simulink model "main"  (R2022a)
settings: Solver=FixedStepDiscrete  StartTime=0.0  StopTime=Inf  FixedStep=(50e-6)-(sim_en*4.995e-5)  RelTol=1e-3  EnableMultiTasking=on
model workspace (MAT data in the model file):
  Param : Simulink.Parameter (value not decoded)
  ac_ok : Simulink.Signal (value not decoded)
  ac_ok_120 : Simulink.Signal (value not decoded)
  bulk_voltage : Simulink.Signal (value not decoded)
  burstduty_integ_max : Simulink.Signal (value not decoded)
  burstduty_integ_min : Simulink.Signal (value not decoded)
  burstduty_ki : Simulink.Signal (value not decoded)
  burstduty_kp : Simulink.Signal (value not decoded)
  calib_ok : Simulink.Signal (value not decoded)
  can_addr1 : Simulink.Signal (value not decoded)
  can_addr2 : Simulink.Signal (value not decoded)
  can_addr3 : Simulink.Signal (value not decoded)
  can_addr4 : Simulink.Signal (value not decoded)
  can_data_rx : Simulink.Signal (value not decoded)
  can_data_tx : Simulink.Signal (value not decoded)
  can_timeout_120 : Simulink.Signal (value not decoded)
  chksum_scircv : Simulink.Signal (value not decoded)
  clllc_en_120 : Simulink.Signal (value not decoded)
  clllc_fault_120 : Simulink.Signal (value not decoded)
  clllc_ok_120 : Simulink.Signal (value not decoded)
  cmpss1h : Simulink.Signal (value not decoded)
  cmpss1l : Simulink.Signal (value not decoded)
  cmpss2h : Simulink.Signal (value not decoded)
  cmpss2l : Simulink.Signal (value not decoded)
  cmpss3h : Simulink.Signal (value not decoded)
  cmpss3l : Simulink.Signal (value not decoded)
  cmpss4h : Simulink.Signal (value not decoded)
  cmpss4l : Simulink.Signal (value not decoded)
  cmpss5h : Simulink.Signal (value not decoded)
  cmpss5l : Simulink.Signal (value not decoded)
  cmpss6h : Simulink.Signal (value not decoded)
  cmpss6l : Simulink.Signal (value not decoded)
  cmpss7h : Simulink.Signal (value not decoded)
  cmpss7l : Simulink.Signal (value not decoded)
  cmpss8h : Simulink.Signal (value not decoded)
  cmpss8l : Simulink.Signal (value not decoded)
  cnt_idle : Simulink.Signal (value not decoded)
  cnt_orps : Simulink.Signal (value not decoded)
  cnt_scircv : Simulink.Signal (value not decoded)
  cnt_scixmt : Simulink.Signal (value not decoded)
  cnt_scixmt_func : Simulink.Signal (value not decoded)
  cnt_temp_mux : Simulink.Signal (value not decoded)
  cnt_vdroop : Simulink.Signal (value not decoded)
  config_ok : Simulink.Signal (value not decoded)
  control_en : Simulink.Signal (value not decoded)
  cp_ready_120 : Simulink.Signal (value not decoded)
  d2d_en : Simulink.Signal (value not decoded)
  dchg_off : Simulink.Signal (value not decoded)
  debug_dacb : Simulink.Signal (value not decoded)
  debug_dacc : Simulink.Signal (value not decoded)
  debug_msg1 : Simulink.Signal (value not decoded)
  debug_msg2 : Simulink.Signal (value not decoded)
  debug_msg3 : Simulink.Signal (value not decoded)
  debug_msg4 : Simulink.Signal (value not decoded)
  debug_msg5 : Simulink.Signal (value not decoded)
  debug_msg6 : Simulink.Signal (value not decoded)
  dir_v2g : Simulink.Signal (value not decoded)
  eoss_llc1 : Simulink.Signal (value not decoded)
  eoss_llc2 : Simulink.Signal (value not decoded)
  eoss_orps : Simulink.Signal (value not decoded)
  fault_ocp : Simulink.Signal (value not decoded)
  fault_otp : Simulink.Signal (value not decoded)
  fault_ovp : Simulink.Signal (value not decoded)
  fut_en : Simulink.Signal (value not decoded)
  fwd_en_120 : Simulink.Signal (value not decoded)
  gain_llc1_sec_idc : Simulink.Signal (value not decoded)
  gain_llc1_temp_sr : Simulink.Signal (value not decoded)
  gain_llc2_sec_idc : Simulink.Signal (value not decoded)
  gain_vbat : Simulink.Signal (value not decoded)
  gain_vbulk : Simulink.Signal (value not decoded)
  gain_vout : Simulink.Signal (value not decoded)
  input_current_phasea : Simulink.Signal (value not decoded)
  input_current_phaseb : Simulink.Signal (value not decoded)
  input_current_phasec : Simulink.Signal (value not decoded)
  input_freq : Simulink.Signal (value not decoded)
  input_power : Simulink.Signal (value not decoded)
  input_voltage_phasea : Simulink.Signal (value not decoded)
  input_voltage_phaseb : Simulink.Signal (value not decoded)
  input_voltage_phasec : Simulink.Signal (value not decoded)
  ishare_arbiter : Simulink.Signal (value not decoded)
  ishare_thresh : Simulink.Signal (value not decoded)
  led_g : Simulink.Signal (value not decoded)
  led_r : Simulink.Signal (value not decoded)
  led_y : Simulink.Signal (value not decoded)
  llc1_burst_integ : Simulink.Signal (value not decoded)
  llc1_burstduty_buffer : Simulink.Signal (value not decoded)
  llc1_pfm_error : Simulink.Signal (value not decoded)
  llc1_pfm_integ : Simulink.Signal (value not decoded)
  llc1_pfm_prop : Simulink.Signal (value not decoded)
  llc1_pri_idc : Simulink.Signal (value not decoded)
  llc1_ps_buffer : Simulink.Signal (value not decoded)
  llc1_pspwm_error : Simulink.Signal (value not decoded)
  llc1_pspwm_integ : Simulink.Signal (value not decoded)
  llc1_pspwm_prop : Simulink.Signal (value not decoded)
  llc1_sec_idc : Simulink.Signal (value not decoded)
  llc1_temp_sr : Simulink.Signal (value not decoded)
  llc1_ts_tbctr_buffer : Simulink.Signal (value not decoded)
  llc2_burst_integ : Simulink.Signal (value not decoded)
  llc2_burstduty_buffer : Simulink.Signal (value not decoded)
  llc2_en : Simulink.Signal (value not decoded)
  llc2_en_buffer : Simulink.Signal (value not decoded)
  llc2_pfm_error : Simulink.Signal (value not decoded)
  llc2_pfm_integ : Simulink.Signal (value not decoded)
  llc2_pfm_prop : Simulink.Signal (value not decoded)
  llc2_pri_idc : Simulink.Signal (value not decoded)
  llc2_ps_buffer : Simulink.Signal (value not decoded)
  llc2_pspwm_error : Simulink.Signal (value not decoded)
  llc2_pspwm_integ : Simulink.Signal (value not decoded)
  llc2_pspwm_prop : Simulink.Signal (value not decoded)
  llc2_sec_idc : Simulink.Signal (value not decoded)
  llc2_temp_sr : Simulink.Signal (value not decoded)
  llc2_ts_tbctr_buffer : Simulink.Signal (value not decoded)
  loop_adcint : Simulink.Signal (value not decoded)
  loop_control : Simulink.Signal (value not decoded)
  loop_idle : Simulink.Signal (value not decoded)
  mid_bulk_voltage : Simulink.Signal (value not decoded)
  mode_120 : Simulink.Signal (value not decoded)
  mode_cc_cv : Simulink.Signal (value not decoded)
  myParam : mpt.Parameter (value not decoded)
  obc_ok_120 : Simulink.Signal (value not decoded)
  offset_llc1_sec_idc : Simulink.Signal (value not decoded)
  offset_llc1_temp_sr : Simulink.Signal (value not decoded)
  offset_llc2_sec_idc : Simulink.Signal (value not decoded)
  offset_vbat : Simulink.Signal (value not decoded)
  offset_vbulk : Simulink.Signal (value not decoded)
  offset_vout : Simulink.Signal (value not decoded)
  openloop_en : Simulink.Signal (value not decoded)
  openloop_fault_en : Simulink.Signal (value not decoded)
  ot_fault_120 : Simulink.Signal (value not decoded)
  pfc_en : Simulink.Signal (value not decoded)
  pfc_en_120 : Simulink.Signal (value not decoded)
  pfc_fw_revision : Simulink.Signal (value not decoded)
  pfc_fw_revision_bootloader : Simulink.Signal (value not decoded)
  pfc_fw_revision_debug : Simulink.Signal (value not decoded)
  pfc_ok : Simulink.Signal (value not decoded)
  pfc_ok_120 : Simulink.Signal (value not decoded)
  pfm_a0 : Simulink.Signal (value not decoded)
  pfm_a1 : Simulink.Signal (value not decoded)
  pfm_integ_max : Simulink.Signal (value not decoded)
  pfm_integ_min : Simulink.Signal (value not decoded)
  pfm_ki : Simulink.Signal (value not decoded)
  pfm_kp : Simulink.Signal (value not decoded)
  pri_fut_en : Simulink.Signal (value not decoded)
  pri_fut_en_buffer : Simulink.Signal (value not decoded)
  pri_halfbridge_en : Simulink.Signal (value not decoded)
  pri_halfbridge_en_buffer : Simulink.Signal (value not decoded)
  pspwm_integ_max : Simulink.Signal (value not decoded)
  pspwm_integ_min : Simulink.Signal (value not decoded)
  pspwm_ki : Simulink.Signal (value not decoded)
  pspwm_kp : Simulink.Signal (value not decoded)
  ref_idclink_max : Simulink.Signal (value not decoded)
  ref_iout : Simulink.Signal (value not decoded)
  ref_iout_calib : Simulink.Signal (value not decoded)
  ref_iout_llc1 : Simulink.Signal (value not decoded)
  ref_iout_llc1_calib : Simulink.Signal (value not decoded)
  ref_iout_llc2 : Simulink.Signal (value not decoded)
  ref_iout_llc2_calib : Simulink.Signal (value not decoded)
  ref_pout : Simulink.Signal (value not decoded)
  ref_ss_llc1 : Simulink.Signal (value not decoded)
  ref_ss_llc2 : Simulink.Signal (value not decoded)
  ref_ss_orps : Simulink.Signal (value not decoded)
  ref_vbat : Simulink.Signal (value not decoded)
  ref_vbat_calib : Simulink.Signal (value not decoded)
  ref_vbulk : Simulink.Signal (value not decoded)
  ref_vbulk_calib : Simulink.Signal (value not decoded)
  ref_vbulk_llc1_calib : Simulink.Signal (value not decoded)
  ref_vbulk_llc2_calib : Simulink.Signal (value not decoded)
  ref_vout : Simulink.Signal (value not decoded)
  ref_vout_calib : Simulink.Signal (value not decoded)
  relay_en : Simulink.Signal (value not decoded)
  reset_flag : Simulink.Signal (value not decoded)
  rev_en_120 : Simulink.Signal (value not decoded)
  runtime_control : Simulink.Signal (value not decoded)
  runtime_idle : Simulink.Signal (value not decoded)
  scircv_buffer : Simulink.Signal (value not decoded)
  scircv_buffer_tmp : Simulink.Signal (value not decoded)
  scircv_buffer_tmp_idx0 : Simulink.Signal (value not decoded)
  scircv_chksum : Simulink.Signal (value not decoded)
  scircv_chksum_ok : Simulink.Signal (value not decoded)
  scircv_parse_ok : Simulink.Signal (value not decoded)
  scixmt_buffer : Simulink.Signal (value not decoded)
  scixmt_chksum : Simulink.Signal (value not decoded)
  scixmt_func : Simulink.Signal (value not decoded)
  scixmt_word0_lsb : Simulink.Signal (value not decoded)
  scixmt_word0_msb : Simulink.Signal (value not decoded)
  scixmt_word1_lsb : Simulink.Signal (value not decoded)
  scixmt_word1_msb : Simulink.Signal (value not decoded)
  scixmt_word2_lsb : Simulink.Signal (value not decoded)
  scixmt_word2_msb : Simulink.Signal (value not decoded)
  scixmt_wr : Simulink.Signal (value not decoded)
  ss_step : Simulink.Signal (value not decoded)
  state_calib : Simulink.Signal (value not decoded)
  state_control : Simulink.Signal (value not decoded)
  state_hkeep : Simulink.Signal (value not decoded)
  status_cmpss : Simulink.Signal (value not decoded)
  status_control : Simulink.Signal (value not decoded)
  status_digin : Simulink.Signal (value not decoded)
  status_digout : Simulink.Signal (value not decoded)
  status_fault : Simulink.Signal (value not decoded)
  status_input : Simulink.Signal (value not decoded)
  status_pfc : Simulink.Signal (value not decoded)
  temp_inlet : Simulink.Signal (value not decoded)
  temp_llc1_fet_hs : Simulink.Signal (value not decoded)
  temp_llc2_fet_hs : Simulink.Signal (value not decoded)
  temp_mux : Simulink.Signal (value not decoded)
  temp_mux_s0 : Simulink.Signal (value not decoded)
  temp_mux_s1 : Simulink.Signal (value not decoded)
  temp_mux_s2 : Simulink.Signal (value not decoded)
  temp_outlet : Simulink.Signal (value not decoded)
  temp_pfc_fet_hsa : Simulink.Signal (value not decoded)
  temp_pfc_fet_hsb : Simulink.Signal (value not decoded)
  temp_pfc_fet_hsc : Simulink.Signal (value not decoded)
  temp_pfc_fet_lsa : Simulink.Signal (value not decoded)
  temp_pfc_fet_lsb : Simulink.Signal (value not decoded)
  temp_pfc_fet_lsc : Simulink.Signal (value not decoded)
  test_mode : Simulink.Signal (value not decoded)
  tfcv_cc : Simulink.Signal (value not decoded)
  tfcv_cc_llc2 : Simulink.Signal (value not decoded)
  tfcv_cv : Simulink.Signal (value not decoded)
  tfcv_sr_en : Simulink.Signal (value not decoded)
  tfv_assert_llc1_pri_idc : Simulink.Signal (value not decoded)
  tfv_assert_llc1_sec_idc : Simulink.Signal (value not decoded)
  tfv_assert_llc1_temp_sr : Simulink.Signal (value not decoded)
  tfv_assert_llc2_pri_idc : Simulink.Signal (value not decoded)
  tfv_assert_llc2_sec_idc : Simulink.Signal (value not decoded)
  tfv_assert_llc2_temp_sr : Simulink.Signal (value not decoded)
  tfv_assert_temp_outlet : Simulink.Signal (value not decoded)
  tfv_assert_vaux_uv : Simulink.Signal (value not decoded)
  tfv_assert_vbat : Simulink.Signal (value not decoded)
  tfv_assert_vbulk : Simulink.Signal (value not decoded)
  tfv_assert_vout : Simulink.Signal (value not decoded)
  tfv_cnt_tz : Simulink.Signal (value not decoded)
  tfv_deassert_llc1_pri_idc : Simulink.Signal (value not decoded)
  tfv_deassert_llc1_sec_idc : Simulink.Signal (value not decoded)
  tfv_deassert_llc1_temp_sr : Simulink.Signal (value not decoded)
  tfv_deassert_llc2_pri_idc : Simulink.Signal (value not decoded)
  tfv_deassert_llc2_sec_idc : Simulink.Signal (value not decoded)
  tfv_deassert_llc2_temp_sr : Simulink.Signal (value not decoded)
  tfv_deassert_temp_outlet : Simulink.Signal (value not decoded)
  tfv_deassert_vaux_uv : Simulink.Signal (value not decoded)
  tfv_deassert_vbat : Simulink.Signal (value not decoded)
  tfv_deassert_vbulk : Simulink.Signal (value not decoded)
  tfv_deassert_vout : Simulink.Signal (value not decoded)
  tfv_llc1_pri_idc : Simulink.Signal (value not decoded)
  tfv_llc1_sec_idc : Simulink.Signal (value not decoded)
  tfv_llc1_temp_sr : Simulink.Signal (value not decoded)
  tfv_llc2_pri_idc : Simulink.Signal (value not decoded)
  tfv_llc2_sec_idc : Simulink.Signal (value not decoded)
  tfv_llc2_temp_sr : Simulink.Signal (value not decoded)
  tfv_temp_outlet : Simulink.Signal (value not decoded)
  tfv_vaux_uv : Simulink.Signal (value not decoded)
  tfv_vbat : Simulink.Signal (value not decoded)
  tfv_vbulk : Simulink.Signal (value not decoded)
  tfv_vout : Simulink.Signal (value not decoded)
  timer_1ms : Simulink.Signal (value not decoded)
  tz : Simulink.Signal (value not decoded)
  valve_en : Simulink.Signal (value not decoded)
  vaux : Simulink.Signal (value not decoded)
  vbat : Simulink.Signal (value not decoded)
  vbulk : Simulink.Signal (value not decoded)
  vout : Simulink.Signal (value not decoded)
undefined symbols (not defined in the file or in its folder): CAN_O_INT, CANA_BASE, Down, GPTRIP1SEL, GPTRIP2SEL, TZ1, TZ2, Up
libraries: hdlsllib x159, simulink x100, c2837xDlib x24, c2807xlib x16, c280xlib x13, c2802xlib x12, canmsglib x8, idelinklib_common x2, c2000lib x1, c281xlib x1
(part 4 of 15)

== system main/Control_State_Machine/update_pwm/deadband_selection ==
  Compare To Constant : simulink/Logic and Bit Operations/Compare To Constant  relop===  const=5.0  OutDataTypeStr=boolean
  Compare To Constant1 : simulink/Logic and Bit Operations/Compare To Constant  relop===  const=9.0  OutDataTypeStr=boolean
  Constant1 : Constant  Commented=on  Value=35  OutDataTypeStr=single
  Constant2 : Constant  Value=0.392  OutDataTypeStr=single
  Constant3 : Constant  Value=321  OutDataTypeStr=double
  Data Store Read1 : DataStoreRead  DataStoreName=sr_delay  IndexOptions=Index vector (dialog)  Indices=1  OutputSizes=1
  Data Store Read2 : DataStoreRead  DataStoreName=deadband  IndexOptions=Index vector (dialog)  Indices=1  OutputSizes=1
  Data Store Read3 : DataStoreRead  DataStoreName=state_control  IndexOptions=Index vector (dialog)  Indices=1  OutputSizes=1
  Data Store Read6 : DataStoreRead  DataStoreName=llc1_ts_tbctr  IndexOptions=Index vector (dialog)  Indices=1  OutputSizes=1
  Data Store Write : DataStoreWrite  DataStoreName=sr_delay  IndexOptions=Index vector (dialog)  Indices=1  OutputSizes=1
  OR : Logic  Operator=OR  IconShape=distinctive  AllPortsSameDT=off  OutDataTypeStr=boolean
  Product1 : Product  OutDataTypeStr=single
  Saturation2 : Saturate  UpperLimit=620  LowerLimit=140  OutDataTypeStr=single
  Subtract1 : Sum  Inputs=+-  AccumDataTypeStr=single  OutDataTypeStr=single
  Switch : Switch  Criteria=u2 > Threshold  SaturateOnIntegerOverflow=off  InputSameDT=off
  Switch1 : Switch  Criteria=u2 > Threshold  SaturateOnIntegerOverflow=off  InputSameDT=off
  to_primos : Outport
  to_secmos : Outport  Port=2
  wires:
  Data Store Read3/1 -> Compare To Constant1/1, Compare To Constant/1
  Compare To Constant/1 -> OR/1
  Compare To Constant1/1 -> OR/2
  OR/1 -> Switch1/2, Switch/2
  Data Store Read1/1 -> Switch1/3, Switch/1
  Switch/1 -> to_primos/1
  Switch1/1 -> to_secmos/1
  Data Store Read2/1 -> Switch1/1, Switch/3
  Data Store Read6/1 -> Product1/1
  Constant3/1 -> Subtract1/2
  Constant2/1 -> Product1/2
  Product1/1 -> Subtract1/1
  Subtract1/1 -> Saturation2/1
  Saturation2/1 -> Data Store Write/1

== system main/Control_State_Machine/update_pwm/to_simulated_plant ==
  note: 1) Add Subsystem or Model blocks as valid variant choices.
      | 2) You cannot connect blocks at this level. At simulation, connectivity is automatically
      | determined, based on the active variant and port name matching.
  codegen : Subsystem  VariantControl=sim_en==0
  sim : Subsystem  VariantControl=sim_en==1
  signal_pwm_cllc1 : Outport

== system main/Task_Manager/Tmr_1mS/codegen ==
  Task_1mS : Subsystem  TreatAsAtomicUnit=on  ScheduleAs=Periodic partition  PartitionName=Task1mS  SystemSampleTime=1e-3
      settings: RTWFcnNameOpts=Use subsystem name  RTWFileNameOpts=Use subsystem name

== system main/Task_Manager/Tmr_1mS/sim ==

== system main/Task_Manager/Tmr_1s/codegen ==
  Task_1S : Subsystem  TreatAsAtomicUnit=on  ScheduleAs=Periodic partition  PartitionName=Task1S  SystemSampleTime=1
      settings: RTWFcnNameOpts=Use subsystem name  RTWFileNameOpts=Use subsystem name

== system main/Task_Manager/Tmr_1s/sim ==

== system main/Task_Manager/Tmr_20mS/codegen ==
  Task_20mS : Subsystem  TreatAsAtomicUnit=on  ScheduleAs=Periodic partition  PartitionName=Task20mS  SystemSampleTime=19e-3
      settings: RTWFcnNameOpts=Use subsystem name  RTWFileNameOpts=Use subsystem name

== system main/Task_Manager/Tmr_20mS/sim ==

== system main/Task_Manager/idle/cnt_idle ==
  function : TriggerPort  TriggerType=function-call  VariantControl=Variant
  Data Store Read : DataStoreRead  DataStoreName=cnt_idle  IndexOptions=Index vector (dialog)  Indices=1  OutputSizes=1
  If : If  IfExpression=u1 < 5
  cnt_idle : Subsystem  TreatAsAtomicUnit=on
  cnt_idle_sat : Subsystem  TreatAsAtomicUnit=on
  wires:
  Data Store Read/1 -> If/1
  If/1 -> cnt_idle/Action
  If/2 -> cnt_idle_sat/Action

== system main/Task_Manager/idle/idle_task ==
  sim_digin : Inport
  function : TriggerPort  TriggerType=function-call  VariantControl=Variant
  Data Store Read : DataStoreRead  DataStoreName=cnt_idle  IndexOptions=Index vector (dialog)  Indices=1  OutputSizes=1
  Switch Case : SwitchCase  CaseConditions={0,1,2,3,4,5}
  calib : Subsystem  TreatAsAtomicUnit=on
  comm_npc : Subsystem  Commented=on  TreatAsAtomicUnit=on
  debug_dac : Subsystem  Commented=on  TreatAsAtomicUnit=on
  debug_uart1 : Subsystem  Commented=on  TreatAsAtomicUnit=on
  hkeep : Subsystem  TreatAsAtomicUnit=on
  status : Subsystem  TreatAsAtomicUnit=on
  uartx : Subsystem  Commented=on  TreatAsAtomicUnit=on
  watchdog : Subsystem  TreatAsAtomicUnit=on
  sim_digout : Outport
  wires:
  Switch Case/1 -> watchdog/Action
  Switch Case/3 -> hkeep/Action
  Switch Case/5 -> comm_npc/Action
  Switch Case/6 -> debug_dac/Action
  status/1(sim_digout) -> sim_digout/1
  Switch Case/4 -> status/Action
  Data Store Read/1 -> Switch Case/1
  Switch Case/2 -> calib/Action
  sim_digin/1 -> status/1(sim_digin)

== system main/Task_Manager/init/codegen ==
  init : Subsystem
      settings: RTWSystemCode=Inline  RTWFcnNameOpts=Use subsystem name  RTWFileNameOpts=Use subsystem name

== system main/Task_Manager/init/sim ==

== system main/interrupt_adcd/burst_control/burst/disPulse ==
  note: EPwm1Regs.AQCSFRC.bit.CSFA = 0b1; //force low
      | EPwm1Regs.AQCSFRC.bit.CSFB = 0b1; //force low
      | EPwm2Regs.AQCSFRC.bit.CSFA = 0b1; //force low
      | EPwm2Regs.AQCSFRC.bit.CSFB = 0b1; //force low
      |
      | EPwm7Regs.AQCSFRC.bit.CSFA = 0b1; //force low
      | EPwm7Regs.AQCSFRC.bit.CSFB = 0b1; //force low
      | EPwm8Regs.AQCSFRC.bit.CSFA = 0b1; //force low
      | EPwm8Regs.AQCSFRC.bit.CSFB = 0b1; //force low
  f : TriggerPort  TriggerType=function-call  VariantControl=(inherit)
      settings: CopyFcn=Stateflow.SLINSF.SimulinkMan.removeBlockPreDeleteFcn  PreDeleteFcn=Stateflow.SLINSF.SimulinkMan.unsafePredeleteFcn
  System Outputs1 : Subsystem  mask(System Outputs){ShowInLibBrowser=0}
      mask prompts: ShowInLibBrowser "Simulink:masks:CustCodeMaskParam1_MP"
      settings: CopyFcn=cccopyfcn(gcb)  OpenFcn=ccopenfcn('System Outputs Function')
      mask Help: eval('feval(''rtwprivate'',''rtwhelpview'',''rtw_sys_outputs_block'')');
      mask DialogControl ShowInLibBrowser Prompt: Mask Parameter 1:
      mask Display: disp('System\nOutputs');

== system main/interrupt_adcd/burst_control/burst/disPwm ==
  note: EPwm1Regs.AQCSFRC.bit.CSFA = 0b1; //force low
      | EPwm1Regs.AQCSFRC.bit.CSFB = 0b1; //force low
      | EPwm2Regs.AQCSFRC.bit.CSFA = 0b1; //force low
      | EPwm2Regs.AQCSFRC.bit.CSFB = 0b1; //force low
      | EPwm7Regs.AQCSFRC.bit.CSFA = 0b1; //force low
      | EPwm7Regs.AQCSFRC.bit.CSFB = 0b1; //force low
      | EPwm8Regs.AQCSFRC.bit.CSFA = 0b1; //force low
      | EPwm8Regs.AQCSFRC.bit.CSFB = 0b1; //force low
  f : TriggerPort  TriggerType=function-call  VariantControl=(inherit)
      settings: CopyFcn=Stateflow.SLINSF.SimulinkMan.removeBlockPreDeleteFcn  PreDeleteFcn=Stateflow.SLINSF.SimulinkMan.unsafePredeleteFcn
  System Outputs1 : Subsystem  mask(System Outputs){ShowInLibBrowser=0}
      mask prompts: ShowInLibBrowser "Simulink:masks:CustCodeMaskParam1_MP"
      settings: CopyFcn=cccopyfcn(gcb)  OpenFcn=ccopenfcn('System Outputs Function')
      mask Help: eval('feval(''rtwprivate'',''rtwhelpview'',''rtw_sys_outputs_block'')');
      mask DialogControl ShowInLibBrowser Prompt: Mask Parameter 1:
      mask Display: disp('System\nOutputs');

== system main/interrupt_adcd/burst_control/burst/enPulse ==
  f : TriggerPort  TriggerType=function-call  VariantControl=(inherit)
      settings: CopyFcn=Stateflow.SLINSF.SimulinkMan.removeBlockPreDeleteFcn  PreDeleteFcn=Stateflow.SLINSF.SimulinkMan.unsafePredeleteFcn
  Data Store Read2 : DataStoreRead  DataStoreName=state_control  IndexOptions=Index vector (dialog)  Indices=1  OutputSizes=1
  Forward : Subsystem  TreatAsAtomicUnit=on
  If1 : If  IfExpression=(u1==3 | u1==8)  ElseIfExpressions=(u1==5 | u1==9)
  Reverse : Subsystem  TreatAsAtomicUnit=on
  wires:
  If1/2 -> Reverse/Action
  If1/1 -> Forward/Action
  Data Store Read2/1 -> If1/1

== system main/interrupt_adcd/get_adc/adc_variant_subsystem ==
  note: 1) Add Subsystem or Model blocks as valid variant choices.
      | 2) You cannot connect blocks at this level. At simulation, connectivity is automatically
      | determined, based on the active variant and port name matching.
  note: ADCA:
      | llc1_sec_idc
      | llc1_pri_idc
      | vout
  note: ADCB :
      | vaux
      | vbulk
      | temp_mux
  sim_adca : Inport
  sim_adcb : Inport  Port=2
  codegen : Subsystem  VariantControl=sim_en==0
  sim : Subsystem  VariantControl=sim_en==1

== system main/interrupt_canrx/canrx_variant_subsystem/codegen ==
  Function-Call Generator2 : simulink/Ports & Subsystems/Function-Call Generator  sample_time=-1  numberOfIterations=1  DisallowWideOutput=off
  can_rcv : Subsystem  TreatAsAtomicUnit=on
  wires:
  Function-Call Generator2/1 -> can_rcv/Trigger

== system main/interrupt_canrx/canrx_variant_subsystem/sim ==
  sim_canrx : Inport
  Data Store Write1 : DataStoreWrite  DataStoreName=f32BurstDuty1  IndexOptions=Index vector (dialog)  Indices=1  OutputSizes=1
  Data Store Write2 : DataStoreWrite  DataStoreName=f32PhaseShift1  IndexOptions=Index vector (dialog)  Indices=1  OutputSizes=1
  Data Store Write3 : DataStoreWrite  DataStoreName=u8OpenLoopEn1  IndexOptions=Index vector (dialog)  Indices=1  OutputSizes=1
  Data Store Write5 : DataStoreWrite  DataStoreName=f32FreqPeriod1  IndexOptions=Index vector (dialog)  Indices=1  OutputSizes=1
  Demux : Demux
  wires:
  sim_canrx/1 -> Demux/1
  Demux/2 -> Data Store Write5/1
  Demux/3 -> Data Store Write2/1
  Demux/4 -> Data Store Write1/1
  Demux/1 -> Data Store Write3/1

== system main/Control_State_Machine/Control_Loop/control/configPowerLimitG2v/If Action Subsystem ==
  ref_vbat : Inport
  ref_iout : Inport  Port=2
  Action Port : ActionPort
  Constant : Constant  Value=2  OutDataTypeStr=uint16
  Divide : Product  Inputs=*/  OutDataTypeStr=uint16
  Product : Product
  Saturation : Saturate  UpperLimit=30000  LowerLimit=0
  ref_pout : Outport
  wires:
  ref_vbat/1 -> Product/1
  ref_iout/1 -> Product/2
  Product/1 -> Saturation/1
  Saturation/1 -> Divide/1
  Divide/1 -> ref_pout/1
  Constant/1 -> Divide/2

== system main/Control_State_Machine/Control_Loop/control/configPowerLimitG2v/If Action Subsystem2 ==
  Action Port : ActionPort
  Constant : Constant  Value=15000  OutDataTypeStr=uint16
  ref_pout : Outport
  wires:
  Constant/1 -> ref_pout/1

== system main/Control_State_Machine/Control_Loop/control/configSr/configXbarEpwmtrip ==
  note: 1) Add Subsystem or Model blocks as valid variant choices.
      | 2) You cannot connect blocks at this level. At simulation, connectivity is automatically
      | determined, based on the active variant and port name matching.
  dir_v2g : Inport
  codegen : Subsystem  VariantControl=sim_en==0
  sim : Subsystem  VariantControl=sim_en==1

== system main/Control_State_Machine/Control_Loop/control/disClb/System Outputs1 ==

== system main/Control_State_Machine/Control_Loop/control/disPwm/System Outputs1 ==

== system main/Control_State_Machine/Control_Loop/control/disableSR/Forward ==
  note: EPwm7Regs.AQCSFRC.bit.CSFA = 0b1; //force low
      | EPwm7Regs.AQCSFRC.bit.CSFB = 0b1; //force low
      | EPwm8Regs.AQCSFRC.bit.CSFA = 0b1; //force low
      | EPwm8Regs.AQCSFRC.bit.CSFB = 0b1; //force low
  Action Port : ActionPort  ActionPortLabel=if((u1==3 | u1==8))
  System Outputs1 : Subsystem  mask(System Outputs){ShowInLibBrowser=0}
      mask prompts: ShowInLibBrowser "Simulink:masks:CustCodeMaskParam1_MP"
      settings: CopyFcn=cccopyfcn(gcb)  OpenFcn=ccopenfcn('System Outputs Function')
      mask Help: eval('feval(''rtwprivate'',''rtwhelpview'',''rtw_sys_outputs_block'')');
      mask DialogControl ShowInLibBrowser Prompt: Mask Parameter 1:
      mask Display: disp('System\nOutputs');

== system main/Control_State_Machine/Control_Loop/control/disableSR/Reverse ==
  note: EPwm1Regs.AQCSFRC.bit.CSFA = 0b1; //force low
      | EPwm1Regs.AQCSFRC.bit.CSFB = 0b1; //force low
      | EPwm2Regs.AQCSFRC.bit.CSFA = 0b1; //force low
      | EPwm2Regs.AQCSFRC.bit.CSFB = 0b1; //force low
  Action Port : ActionPort  ActionPortLabel=elseif((u1==5 | u1==9))
  System Outputs1 : Subsystem  mask(System Outputs){ShowInLibBrowser=0}
      mask prompts: ShowInLibBrowser "Simulink:masks:CustCodeMaskParam1_MP"
      settings: CopyFcn=cccopyfcn(gcb)  OpenFcn=ccopenfcn('System Outputs Function')
      mask Help: eval('feval(''rtwprivate'',''rtwhelpview'',''rtw_sys_outputs_block'')');
      mask DialogControl ShowInLibBrowser Prompt: Mask Parameter 1:
      mask Display: disp('System\nOutputs');

== system main/Control_State_Machine/Control_Loop/control/enableSR/Forward ==
  note: EPwm7Regs.AQCSFRC.bit.CSFA = 0b0; //force disabled
      | EPwm7Regs.AQCSFRC.bit.CSFB = 0b0; //force disabled
      | EPwm8Regs.AQCSFRC.bit.CSFA = 0b0; //force disabled
      | EPwm8Regs.AQCSFRC.bit.CSFB = 0b0; //force disabled
  Action Port : ActionPort  ActionPortLabel=if((u1==3 | u1==8))
  System Outputs1 : Subsystem  mask(System Outputs){ShowInLibBrowser=0}
      mask prompts: ShowInLibBrowser "Simulink:masks:CustCodeMaskParam1_MP"
      settings: CopyFcn=cccopyfcn(gcb)  OpenFcn=ccopenfcn('System Outputs Function')
      mask Help: eval('feval(''rtwprivate'',''rtwhelpview'',''rtw_sys_outputs_block'')');
      mask DialogControl ShowInLibBrowser Prompt: Mask Parameter 1:
      mask Display: disp('System\nOutputs');

== system main/Control_State_Machine/Control_Loop/control/enableSR/Reverse ==
  note: EPwm1Regs.AQCSFRC.bit.CSFA = 0b0; //force disabled
      | EPwm1Regs.AQCSFRC.bit.CSFB = 0b0; //force disabled
      | EPwm2Regs.AQCSFRC.bit.CSFA = 0b0; //force disabled
      | EPwm2Regs.AQCSFRC.bit.CSFB = 0b0; //force disabled
  Action Port : ActionPort  ActionPortLabel=elseif((u1==5 | u1==9))
  System Outputs1 : Subsystem  mask(System Outputs){ShowInLibBrowser=0}
      mask prompts: ShowInLibBrowser "Simulink:masks:CustCodeMaskParam1_MP"
      settings: CopyFcn=cccopyfcn(gcb)  OpenFcn=ccopenfcn('System Outputs Function')
      mask Help: eval('feval(''rtwprivate'',''rtwhelpview'',''rtw_sys_outputs_block'')');
      mask DialogControl ShowInLibBrowser Prompt: Mask Parameter 1:
      mask Display: disp('System\nOutputs');

== system main/Control_State_Machine/Control_Loop/control/tzClear/System Outputs ==

== system main/Control_State_Machine/update_pwm/to_simulated_plant/codegen ==
  signal_pwm_cllc1 : Outport

== system main/Control_State_Machine/update_pwm/to_simulated_plant/sim ==
  Data Store Read3 : DataStoreRead  DataStoreName=llc1_ps  IndexOptions=Index vector (dialog)  Indices=1  OutputSizes=1
  Data Store Read4 : DataStoreRead  DataStoreName=llc1_ts_tbctr  IndexOptions=Index vector (dialog)  Indices=1  OutputSizes=1
  Mux2 : Mux  Inputs=2
  signal_pwm_cllc1 : Outport
  wires:
  Data Store Read4/1 -> Mux2/1
  Data Store Read3/1 -> Mux2/2
  Mux2/1 -> signal_pwm_cllc1/1

== system main/Task_Manager/Tmr_1mS/codegen/Task_1mS ==
  Counter_1mS : Subsystem  TreatAsAtomicUnit=on
      settings: RTWSystemCode=Inline
  Function-Call Generator1 : simulink/Ports & Subsystems/Function-Call Generator  sample_time=-1  numberOfIterations=1  DisallowWideOutput=off
  Function-Call Split3 : FunctionCallSplit  NumOutputPorts=2
  GPIO_Handler : Subsystem  TreatAsAtomicUnit=on
      settings: RTWSystemCode=Inline
  wires:
  Function-Call Generator1/1 -> Function-Call Split3/1
  Function-Call Split3/1 -> Counter_1mS/Trigger
  Function-Call Split3/2 -> GPIO_Handler/Trigger

== system main/Task_Manager/Tmr_1s/codegen/Task_1S ==
  Function-Call Generator1 : simulink/Ports & Subsystems/Function-Call Generator  sample_time=-1  numberOfIterations=1  DisallowWideOutput=off
  Function-Call Split3 : FunctionCallSplit  NumOutputPorts=2
  addressing_temp_mux : Subsystem  TreatAsAtomicUnit=on
      settings: RTWSystemCode=Inline
  cnt_temp_mux : Subsystem  TreatAsAtomicUnit=on
      settings: RTWSystemCode=Inline
  wires:
  Function-Call Split3/2 -> addressing_temp_mux/Trigger
  Function-Call Split3/1 -> cnt_temp_mux/Trigger
  Function-Call Generator1/1 -> Function-Call Split3/1

== system main/Task_Manager/Tmr_20mS/codegen/Task_20mS ==
  Function-Call Generator1 : simulink/Ports & Subsystems/Function-Call Generator  sample_time=-1  numberOfIterations=1  DisallowWideOutput=off
  Function-Call Split1 : FunctionCallSplit  NumOutputPorts=2
  Rx_Handler : Subsystem  TreatAsAtomicUnit=on
  Tx_Handler : Subsystem  TreatAsAtomicUnit=on
  wires:
  Function-Call Split1/2 -> Tx_Handler/Trigger
  Function-Call Split1/1 -> Rx_Handler/Trigger
  Function-Call Generator1/1 -> Function-Call Split1/1

== system main/Task_Manager/idle/cnt_idle/cnt_idle ==
  Action Port : ActionPort  ActionPortLabel=if(u1 < 5)
  Add : Sum
  Constant : Constant  OutDataTypeStr=uint16
  Data Store Read1 : DataStoreRead  DataStoreName=cnt_idle  IndexOptions=Index vector (dialog)  Indices=1  OutputSizes=1
  Data Store Write : DataStoreWrite  DataStoreName=cnt_idle  IndexOptions=Index vector (dialog)  Indices=1  OutputSizes=1
  wires:
  Data Store Read1/1 -> Add/1
  Add/1 -> Data Store Write/1
  Constant/1 -> Add/2

== system main/Task_Manager/idle/cnt_idle/cnt_idle_sat ==
  Action Port : ActionPort  ActionPortLabel=else
  Constant : Constant  Value=0  OutDataTypeStr=uint16
  Data Store Write : DataStoreWrite  DataStoreName=cnt_idle  IndexOptions=Index vector (dialog)  Indices=1  OutputSizes=1
  wires:
  Constant/1 -> Data Store Write/1

== system main/Task_Manager/idle/idle_task/calib ==
  note: Note:
      | calibrates one time for:
      | references
      | protection levels
      | unless change in reference during run
      | time is initiated (test purposes only)
  Action Port : ActionPort  ActionPortLabel=case [ 1 ]:
  calib : Stateflow chart  TreatAsAtomicUnit=on

== system main/Task_Manager/idle/idle_task/comm_npc ==
  Action Port : ActionPort  ActionPortLabel=case [ 4 ]:
  comm_npc : Stateflow chart  TreatAsAtomicUnit=on

== system main/Task_Manager/idle/idle_task/debug_dac ==
  Action Port : ActionPort  ActionPortLabel=case [ 5 ]:
  DAC : c2837xDlib/DAC  Commented=on  channel=B  saturate=off
      settings: SourceProductBaseCode=TIC2000
  DAC1 : c2837xDlib/DAC  Commented=on  channel=C  saturate=off
      settings: SourceProductBaseCode=TIC2000

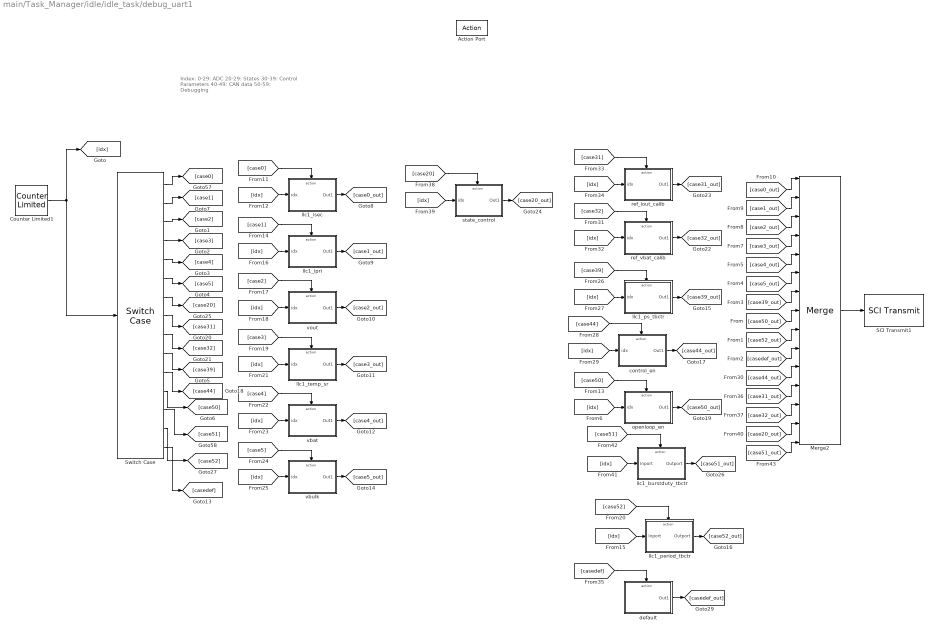
== system main/Task_Manager/idle/idle_task/debug_uart1 ==
  note: Index:
      | 0-29: ADC
      | 20-29: States
      | 30-39: Control Parameters
      | 40-49: CAN data
      | 50-59: Debugging
  Action Port : ActionPort
  Counter Limited1 : simulink/Sources/Counter Limited  uplimit=76  tsamp=-1
  Merge2 : Merge  Inputs=15
  SCI Transmit1 : c280xlib/SCI Transmit  sciModule=A  dataHead='E'  dataTail='S'  blockingMode=on  outputStatus=off
  Switch Case : SwitchCase  CaseConditions={0,1,2,3,4,5,20,31,32,39,44,50,51,52}
  control_en : Subsystem  TreatAsAtomicUnit=on
  default : Subsystem  TreatAsAtomicUnit=on
  llc1_burstduty_tbctr : Subsystem  TreatAsAtomicUnit=on
  llc1_ipri : Subsystem  TreatAsAtomicUnit=on
  llc1_isec : Subsystem  TreatAsAtomicUnit=on
  llc1_period_tbctr : Subsystem  TreatAsAtomicUnit=on
  llc1_ps_tbctr : Subsystem  TreatAsAtomicUnit=on
  llc1_temp_sr : Subsystem  TreatAsAtomicUnit=on
  openloop_en : Subsystem  TreatAsAtomicUnit=on
  ref_iout_calib : Subsystem  TreatAsAtomicUnit=on
  ref_vbat_calib : Subsystem  TreatAsAtomicUnit=on
  state_control : Subsystem  TreatAsAtomicUnit=on
  vbat : Subsystem  TreatAsAtomicUnit=on
  vbulk : Subsystem  TreatAsAtomicUnit=on
  vout : Subsystem  TreatAsAtomicUnit=on
  wires:
  [case51_out] -> Merge2/15
  Switch Case/14 -> [case52]
  [case51] -> llc1_burstduty_tbctr/Action
  [idx] -> llc1_burstduty_tbctr/1(Inport)
  llc1_burstduty_tbctr/1(Outport) -> [case51_out]
  [casedef_out] -> Merge2/10
  [case32_out] -> Merge2/13
  [idx] -> llc1_isec/1(idx)
  [case39_out] -> Merge2/7
  openloop_en/1(Out1) -> [case50_out]
  Merge2/1 -> SCI Transmit1/1
  Counter Limited1/1 -> [idx], Switch Case/1
  [case1_out] -> Merge2/2
  llc1_isec/1(Out1) -> [case0_out]
  Switch Case/10 -> [case39]
  Switch Case/2 -> [case1]
  [idx] -> ref_vbat_calib/1(idx)
  Switch Case/5 -> [case4]
  [idx] -> llc1_ps_tbctr/1(idx)
  default/1(Out1) -> [casedef_out]
  Switch Case/4 -> [case3]
  [case44] -> control_en/Action
  [case39] -> llc1_ps_tbctr/Action
  Switch Case/3 -> [case2]
  [case50_out] -> Merge2/8
  [idx] -> openloop_en/1(idx)
  [casedef] -> default/Action
  [idx] -> vbat/1(idx)
  [case2] -> vout/Action
  llc1_ipri/1(Out1) -> [case1_out]
  llc1_ps_tbctr/1(Out1) -> [case39_out]
  [case3] -> llc1_temp_sr/Action
  [case31_out] -> Merge2/12
  [case0_out] -> Merge2/1
  llc1_period_tbctr/1(Outport) -> [case52_out]
  vout/1(Out1) -> [case2_out]
  [case0] -> llc1_isec/Action
  [idx] -> llc1_temp_sr/1(idx)
  [idx] -> llc1_ipri/1(idx)
  [case4] -> vbat/Action
  [case20_out] -> Merge2/14
  llc1_temp_sr/1(Out1) -> [case3_out]
  [case50] -> openloop_en/Action
  [case2_out] -> Merge2/3
  vbulk/1(Out1) -> [case5_out]
  vbat/1(Out1) -> [case4_out]
  [idx] -> vbulk/1(idx)
  Switch Case/8 -> [case31]
  [idx] -> llc1_period_tbctr/1(Inport)
  [case52_out] -> Merge2/9
  [idx] -> control_en/1(idx)
  [case5] -> vbulk/Action
  Switch Case/6 -> [case5]
  Switch Case/11 -> [case44]
  Switch Case/13 -> [case51]
  [case32] -> ref_vbat_calib/Action
  Switch Case/9 -> [case32]
  [case44_out] -> Merge2/11
  [case5_out] -> Merge2/6
  Switch Case/15 -> [casedef]
  [case3_out] -> Merge2/4
  [case4_out] -> Merge2/5
  [idx] -> ref_iout_calib/1(idx)
  Switch Case/12 -> [case50]
  ref_iout_calib/1(Out1) -> [case31_out]
  [case31] -> ref_iout_calib/Action
  Switch Case/1 -> [case0]
  [idx] -> vout/1(idx)
  [idx] -> state_control/1(idx)
  [case20] -> state_control/Action
  [case1] -> llc1_ipri/Action
  control_en/1(Out1) -> [case44_out]
  [case52] -> llc1_period_tbctr/Action
  ref_vbat_calib/1(Out1) -> [case32_out]
  Switch Case/7 -> [case20]
  state_control/1(Out1) -> [case20_out]

== system main/Task_Manager/idle/idle_task/hkeep ==
  Action Port : ActionPort  ActionPortLabel=case [ 2 ]:
  Function-Call Generator1 : simulink/Ports & Subsystems/Function-Call Generator  sample_time=-1  numberOfIterations=1  DisallowWideOutput=off
  Function-Call Split3 : FunctionCallSplit  NumOutputPorts=2
  tfv : Subsystem  TreatAsAtomicUnit=on
      settings: RTWSystemCode=Inline
  tz : Subsystem  TreatAsAtomicUnit=on
      settings: RTWSystemCode=Inline
  wires:
  Function-Call Split3/1 -> tz/Trigger
  Function-Call Split3/2 -> tfv/Trigger
  Function-Call Generator1/1 -> Function-Call Split3/1

== system main/Task_Manager/idle/idle_task/status ==
  sim_digin : Inport
  Action Port : ActionPort  ActionPortLabel=case [ 3 ]:
  Function-Call Generator : simulink/Ports & Subsystems/Function-Call Generator  sample_time=-1  numberOfIterations=1  DisallowWideOutput=off
  Function-Call Split{,1,3..4} (4 alike) : FunctionCallSplit  NumOutputPorts=2  OutputPortLayout=default
  init : Subsystem  Commented=on  TreatAsAtomicUnit=on
      settings: RTWSystemCode=Inline
  status_control : Subsystem  Commented=on  TreatAsAtomicUnit=on
      settings: RTWSystemCode=Inline
  status_digin : Subsystem  Commented=on  TreatAsAtomicUnit=on
      settings: RTWSystemCode=Inline
  status_digout : Subsystem  Commented=on  TreatAsAtomicUnit=on
      settings: RTWSystemCode=Inline
  status_fault : Subsystem  Commented=on  TreatAsAtomicUnit=on
      settings: RTWSystemCode=Inline
  update_CAN_msg1 : Subsystem  TreatAsAtomicUnit=on
      settings: RTWSystemCode=Inline
  sim_digout : Outport
  wires:
  Function-Call Split3/2 -> status_fault/Trigger
  init/1(sim_digout) -> sim_digout/1
  Function-Call Generator/1 -> Function-Call Split/1
  Function-Call Split3/1 -> Function-Call Split1/1
  Function-Call Split/1 -> Function-Call Split4/1
  sim_digin/1 -> init/1(sim_digin)
  Function-Call Split/2 -> init/Trigger
  Function-Call Split4/2 -> status_control/Trigger
  Function-Call Split4/1 -> Function-Call Split3/1
  Function-Call Split1/2 -> status_digin/Trigger
  Function-Call Split1/1 -> update_CAN_msg1/Trigger

== system main/Task_Manager/idle/idle_task/uartx ==
  Action Port : ActionPort  ActionPortLabel=case [ 4 ]:
  Function-Call Generator1 : simulink/Ports & Subsystems/Function-Call Generator  sample_time=-1  numberOfIterations=1  DisallowWideOutput=off
  Function-Call Split2 : FunctionCallSplit  NumOutputPorts=2
  Function-Call Split4 : FunctionCallSplit  NumOutputPorts=2
  extract_status : Subsystem  TreatAsAtomicUnit=on
  parse : Subsystem  TreatAsAtomicUnit=on
  uart_xmt : Subsystem  TreatAsAtomicUnit=on
  wires:
  Function-Call Split4/1 -> extract_status/Trigger
  Function-Call Split2/1 -> parse/Trigger
  Function-Call Split2/2 -> uart_xmt/Trigger
  Function-Call Split4/2 -> Function-Call Split2/1
  Function-Call Generator1/1 -> Function-Call Split4/1

== system main/Task_Manager/idle/idle_task/watchdog ==
  Action Port : ActionPort  ActionPortLabel=case [ 0 ]:
  Watchdog : c281xlib/Watchdog  resetsrc=Specify via dialog  sample=-1
      settings: SourceProductBaseCode=TIC2000

== system main/Task_Manager/init/codegen/init ==
  Function-Call Generator1 : simulink/Ports & Subsystems/Function-Call Generator  sample_time=-1  numberOfIterations=1  DisallowWideOutput=off
  Function-Call Split{1..3,5} (4 alike) : FunctionCallSplit  NumOutputPorts=2
  cmpss : Subsystem  TreatAsAtomicUnit=on
      settings: RTWSystemCode=Inline
  orps&relay : Subsystem  TreatAsAtomicUnit=on
      settings: RTWSystemCode=Inline
  outputxbar : Subsystem  Commented=on  TreatAsAtomicUnit=on
      settings: RTWSystemCode=Inline
  pwmsync : Subsystem  TreatAsAtomicUnit=on
      settings: RTWSystemCode=Inline
  tztl_clb : Subsystem  Commented=on  TreatAsAtomicUnit=on
      settings: RTWSystemCode=Inline
  wires:
  Function-Call Split5/1 -> cmpss/Trigger
  Function-Call Split5/2 -> Function-Call Split2/1
  Function-Call Split2/1 -> outputxbar/Trigger
  Function-Call Split2/2 -> tztl_clb/Trigger
  Function-Call Split3/2 -> Function-Call Split5/1
  Function-Call Split1/2 -> Function-Call Split3/1
  Function-Call Generator1/1 -> Function-Call Split1/1
  Function-Call Split1/1 -> pwmsync/Trigger
  Function-Call Split3/1 -> orps&relay/Trigger

== system main/interrupt_adcd/burst_control/burst/disPulse/System Outputs1 ==

== system main/interrupt_adcd/burst_control/burst/disPwm/System Outputs1 ==

== system main/interrupt_adcd/burst_control/burst/enPulse/Forward ==
  note: EPwm1Regs.AQCSFRC.bit.CSFA = 0b0; //force disabled
      | EPwm1Regs.AQCSFRC.bit.CSFB = 0b0; //force disabled
      | EPwm2Regs.AQCSFRC.bit.CSFA = 0b0; //force disabled
      | EPwm2Regs.AQCSFRC.bit.CSFB = 0b0; //force disabled
  Action Port : ActionPort  ActionPortLabel=if((u1==3 | u1==8))
  System Outputs1 : Subsystem  mask(System Outputs){ShowInLibBrowser=0}
      mask prompts: ShowInLibBrowser "Simulink:masks:CustCodeMaskParam1_MP"
      settings: CopyFcn=cccopyfcn(gcb)  OpenFcn=ccopenfcn('System Outputs Function')
      mask Help: eval('feval(''rtwprivate'',''rtwhelpview'',''rtw_sys_outputs_block'')');
      mask DialogControl ShowInLibBrowser Prompt: Mask Parameter 1:
      mask Display: disp('System\nOutputs');

== system main/interrupt_adcd/burst_control/burst/enPulse/Reverse ==
  note: EPwm7Regs.AQCSFRC.bit.CSFA = 0b0; //force disabled
      | EPwm7Regs.AQCSFRC.bit.CSFB = 0b0; //force disabled
      | EPwm8Regs.AQCSFRC.bit.CSFA = 0b0; //force disabled
      | EPwm8Regs.AQCSFRC.bit.CSFB = 0b0; //force disabled
  Action Port : ActionPort  ActionPortLabel=elseif((u1==5 | u1==9))
  System Outputs1 : Subsystem  mask(System Outputs){ShowInLibBrowser=0}
      mask prompts: ShowInLibBrowser "Simulink:masks:CustCodeMaskParam1_MP"
      settings: CopyFcn=cccopyfcn(gcb)  OpenFcn=ccopenfcn('System Outputs Function')
      mask Help: eval('feval(''rtwprivate'',''rtwhelpview'',''rtw_sys_outputs_block'')');
      mask DialogControl ShowInLibBrowser Prompt: Mask Parameter 1:
      mask Display: disp('System\nOutputs');

== system main/interrupt_adcd/get_adc/adc_variant_subsystem/codegen ==
  note: D4: T_DD_AD
  sim_adca : Inport
  ADC1 : c2802xlib/ADC  blkParamProc=C2000_Type4  ADCModule=D  samplingMode=Single sample mode  ADCResolution=12-bit (Single-ended input)  useSOC1=SOC5  useSOC2=SOC0_SOC1  SOCAcquisitionWindow=7  SOCTriggerSource=ePWM3_ADCSOCA  SOCInterruptTrigger=No ADCINT  Ts=-1  dType=uint16  postInterrupt=on  interruptSel=ADCINT1  ADCINTContinuous=off  endma=off  chdma=1  conv1=ADCINA0  conv2=ADCINA0 and ADCINB0  conv1_Type4=ADCIN4  conv2_Type4=ADCIN0 and ADCIN1
  Data Store Write1 : DataStoreWrite  DataStoreName=temp_mux  IndexOptions=Index vector (dialog)  Indices=1  OutputSizes=1
  wires:
  ADC1/1 -> Data Store Write1/1

== system main/interrupt_adcd/get_adc/adc_variant_subsystem/sim ==
  sim_adca : Inport
  sim_adcb : Inport  Port=2
  Bus Selector1 : BusSelector  OutputSignals=vbulk,vaux,temp_mux
  Bus Selector2 : BusSelector  OutputSignals=vout,llc1_sec_idc,llc1_pri_idc
  Cast To Single{,1,3..5} (5 alike) : DataTypeConversion  OutDataTypeStr=single  SaturateOnIntegerOverflow=off  RndMeth=Floor
  Data Store Write1 : DataStoreWrite  DataStoreName=llc1_sec_idc  IndexOptions=Index vector (dialog)  Indices=1  OutputSizes=1
  Data Store Write2 : DataStoreWrite  DataStoreName=llc1_pri_idc  IndexOptions=Index vector (dialog)  Indices=1  OutputSizes=1
  Data Store Write23 : DataStoreWrite  DataStoreName=vbulk  IndexOptions=Index vector (dialog)  Indices=1  OutputSizes=1
  Data Store Write25 : DataStoreWrite  DataStoreName=vaux  IndexOptions=Index vector (dialog)  Indices=1  OutputSizes=1
  Data Store Write4 : DataStoreWrite  DataStoreName=vout  IndexOptions=Index vector (dialog)  Indices=1  OutputSizes=1
  Data Store Write6 : DataStoreWrite  DataStoreName=temp_mux  IndexOptions=Index vector (dialog)  Indices=1  OutputSizes=1
  wires:
  [llc1_sec_idc] -> Cast To Single/1
  [llc1_pri_idc] -> Cast To Single1/1
  Bus Selector2/1 -> [vout]  "<vout>"
  Bus Selector2/2 -> [llc1_sec_idc]  "<llc1_sec_idc>"
  Bus Selector2/3 -> [llc1_pri_idc]  "<llc1_pri_idc>"
  sim_adca/1 -> Bus Selector2/1
  sim_adcb/1 -> Bus Selector1/1
  Bus Selector1/1 -> [vbulk]  "<vbulk>"
  Bus Selector1/2 -> [vaux]  "<vaux>"
  [vbulk] -> Cast To Single4/1
  [vaux] -> Cast To Single3/1
  [temp_mux] -> Cast To Single5/1
  Bus Selector1/3 -> [temp_mux]  "<temp_mux>"
  Cast To Single/1 -> Data Store Write1/1
  Cast To Single1/1 -> Data Store Write2/1
  [vout] -> Data Store Write4/1
  Cast To Single3/1 -> Data Store Write25/1
  Cast To Single4/1 -> Data Store Write23/1
  Cast To Single5/1 -> Data Store Write6/1

== system main/interrupt_canrx/canrx_variant_subsystem/codegen/can_rcv ==
  note: Read the CAN Data
  function : TriggerPort  TriggerType=function-call  VariantControl=Variant
  Bitwise AND : simulink/Logic and Bit Operations/Bitwise Operator  logicop=AND  UseBitMask=on  BitMask=hex2dec('0000003F')  BitMaskRealWorld=Stored Integer
  CANA_CAN0INT : idelinklib_common/Memory Copy  Priority=2  copyFrom=Specified source code symbol  copyFromAddressSource=Specify via dialog  copyFromAddress=hex2dec('48108')  copyFromSrcCode=(CANA_BASE + CAN_O_INT)  dataTypeFrom=uint32  dataDimensionFrom=1  useOffsetFrom=off  offsetFromSrc=Specify via dialog  offsetFrom=0  strideFrom=1  copyTo=Output port  copyToAddressSource=Specify via dialog  copyToAddress=hex2dec('00002000')  copyToSrcCode=myVariableDst  dataTypeTo=uint32  useOffsetTo=off  offsetToSrc=Specify via dialog  offsetTo=0  strideTo=1  sampleTime=-1  useInitValue=off  initValueSrc=Specify constant value  initValue=1  initValueSrcCode=myInitValueVariable  useAsMask=off  maskOperator=bitwise AND  useTermValue=off  termValue=1  isRealtimeEnabled=off  emitCCBeforeWrite=off  CCBeforeWrite=/* Custom Code Before Write*/  emitCCAfterWrite=off  CCAfterWrite=/* Custom Code After Write*/  useDMACopy=off  enableBlockingMode=off
      settings: SourceProductBaseCode=ME
  Switch Case : SwitchCase  CaseConditions={10,11,12}  ShowDefaultCase=off
  Switch Case Action Subsystem : Subsystem  TreatAsAtomicUnit=on
  Switch Case Action Subsystem1 : Subsystem  TreatAsAtomicUnit=on
  Switch Case Action Subsystem2 : Subsystem  TreatAsAtomicUnit=on
  wires:
  Switch Case/1 -> Switch Case Action Subsystem/Action
  Switch Case/3 -> Switch Case Action Subsystem2/Action
  Switch Case/2 -> Switch Case Action Subsystem1/Action
  CANA_CAN0INT/1 -> Bitwise AND/1
  Bitwise AND/1 -> Switch Case/1

== system main/Control_State_Machine/Control_Loop/control/configSr/configXbarEpwmtrip/codegen ==
  dir_v2g : Inport
  If : If  IfExpression=(u1==0)  ElseIfExpressions=(u1==1)  ShowElse=off
  g2v_prifullbridge : Subsystem  TreatAsAtomicUnit=on
  v2g_prifullbridge : Subsystem  TreatAsAtomicUnit=on
  wires:
  dir_v2g/1 -> If/1
  If/2 -> v2g_prifullbridge/Action
  If/1 -> g2v_prifullbridge/Action

== system main/Control_State_Machine/Control_Loop/control/configSr/configXbarEpwmtrip/sim ==
  dir_v2g : Inport
  If : If  IfExpression=(u1==0)
  g2v_prifullbridge : Subsystem  TreatAsAtomicUnit=on
  v2g_prifullbridge : Subsystem  TreatAsAtomicUnit=on
  wires:
  If/2 -> v2g_prifullbridge/Action
  dir_v2g/1 -> If/1
  If/1 -> g2v_prifullbridge/Action

== system main/Control_State_Machine/Control_Loop/control/disableSR/Forward/System Outputs1 ==

== system main/Control_State_Machine/Control_Loop/control/disableSR/Reverse/System Outputs1 ==

== system main/Control_State_Machine/Control_Loop/control/enableSR/Forward/System Outputs1 ==

== system main/Control_State_Machine/Control_Loop/control/enableSR/Reverse/System Outputs1 ==

== system main/Task_Manager/Tmr_1mS/codegen/Task_1mS/Counter_1mS ==
  note: Note:
      |  - Worst error of tfv is timer interval (1ms) + twice the execution of supervisory loop
      |  - Effective max count is 65.536 = 2e16*1e-3
  function : TriggerPort  TriggerType=function-call  VariantControl=Variant
  Add : Sum
  Constant : Constant  OutDataTypeStr=uint16
  Data Store Read : DataStoreRead  DataStoreName=timer_1ms  IndexOptions=Index vector (dialog)  Indices=1  OutputSizes=1
  Data Store Write : DataStoreWrite  DataStoreName=timer_1ms  IndexOptions=Index vector (dialog)  Indices=1  OutputSizes=1
  wires:
  Constant/1 -> Add/2
  Add/1 -> Data Store Write/1
  Data Store Read/1 -> Add/1
